simulink model "MF3"  (R2022a)
settings: Solver=VariableStepAuto  StartTime=0.0  StopTime=10.0  RelTol=1e-3
libraries: simulink x8, mbedblockslib x1
settings Model: Creator=FUGAZI  LastModifiedBy=smith

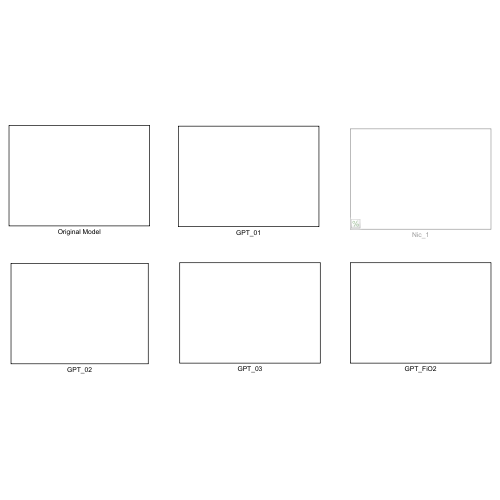
[thumbnail: Simulink's stored preview of the top-level diagram]
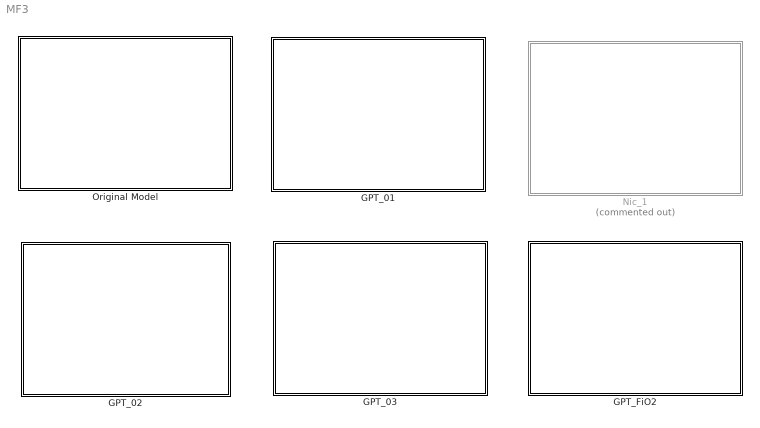
== system MF3 ==
  GPT_01 : Subsystem
  GPT_02 : Subsystem
  GPT_03 : Subsystem
  GPT_FiO2 : Subsystem
  Nic_1 : Subsystem  Commented=on
  Original Model : Subsystem

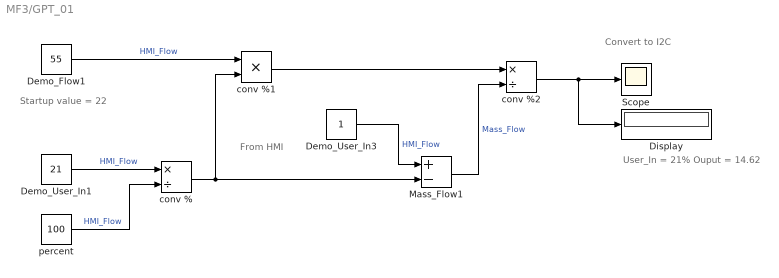
== system MF3/GPT_01 ==
  note: From HMI
  note: Startup value = 22
  note: Convert to I2C
  note: User_In = 21%
      | Ouput = 14.62
  Demo_Flow1 : Constant  Value=55
  Demo_User_In1 : Constant  Value=21
  Demo_User_In3 : Constant
  Display : Display
  Mass_Flow1 : Sum  Inputs=+-
  Scope : Scope
  conv % : Product  Inputs=*/
  conv %1 : Product  Inputs=**
  conv %2 : Product  Inputs=*/
  percent : Constant  Value=100
  wires:
  conv %1/1 -> conv %2/1
  Mass_Flow1/1 -> conv %2/2  "Mass_Flow"
  conv %/1 -> Mass_Flow1/2, conv %1/2
  conv %2/1 -> Display/1, Scope/1
  Demo_Flow1/1 -> conv %1/1  "HMI_Flow"
  Demo_User_In1/1 -> conv %/1  "HMI_Flow"
  percent/1 -> conv %/2  "HMI_Flow"
  Demo_User_In3/1 -> Mass_Flow1/1  "HMI_Flow"

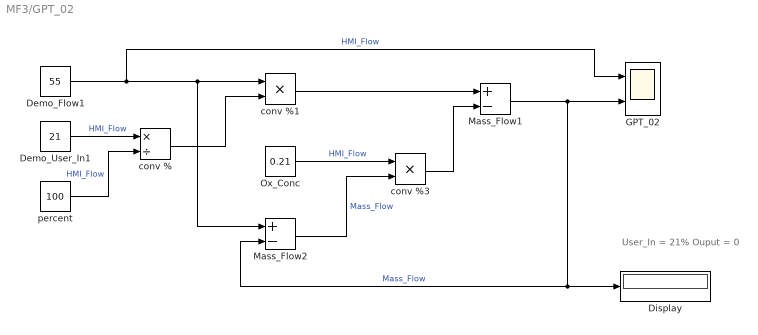
== system MF3/GPT_02 ==
  note: User_In = 21%
      | Ouput = 0
  Demo_Flow1 : Constant  Value=55
  Demo_User_In1 : Constant  Value=21
  Display : Display
  GPT_02 : Scope  NumInputPorts=2
  Mass_Flow1 : Sum  Inputs=+-
  Mass_Flow2 : Sum  Inputs=+-
  Ox_Conc : Constant  Value=0.21
  conv % : Product  Inputs=*/
  conv %1 : Product  Inputs=**
  conv %3 : Product  Inputs=**
  percent : Constant  Value=100
  wires:
  percent/1 -> conv %/2  "HMI_Flow"
  Demo_User_In1/1 -> conv %/1  "HMI_Flow"
  Demo_Flow1/1 -> GPT_02/1, Mass_Flow2/1, conv %1/1  "HMI_Flow"
  conv %/1 -> conv %1/2
  conv %1/1 -> Mass_Flow1/1
  Mass_Flow1/1 -> Display/1, Mass_Flow2/2, GPT_02/2  "Mass_Flow"
  conv %3/1 -> Mass_Flow1/2
  Ox_Conc/1 -> conv %3/1  "HMI_Flow"
  Mass_Flow2/1 -> conv %3/2  "Mass_Flow"

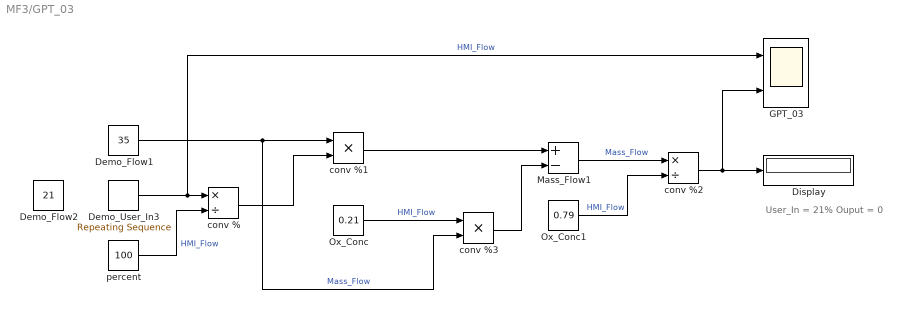
== system MF3/GPT_03 ==
  note: User_In = 21%
      | Ouput = 0
  Demo_Flow1 : Constant  Value=35
  Demo_Flow2 : Constant  Value=21
  Demo_User_In3 : simulink/Sources/Repeating Sequence  rep_seq_t=[0 1 1.1 2 2.1 3 3.1 4 4.1]  rep_seq_y=[21 21 65 65 35 35 45 45 21]
  Display : Display
  GPT_03 : Scope  NumInputPorts=2
  Mass_Flow1 : Sum  Inputs=+-
  Ox_Conc : Constant  Value=0.21
  Ox_Conc1 : Constant  Value=0.79
  conv % : Product  Inputs=*/
  conv %1 : Product  Inputs=**
  conv %2 : Product  Inputs=*/
  conv %3 : Product  Inputs=**
  percent : Constant  Value=100
  wires:
  Demo_Flow1/1 -> conv %3/2, conv %1/1  "Mass_Flow"
  conv %3/1 -> Mass_Flow1/2
  Demo_User_In3/1 -> GPT_03/1, conv %/1  "HMI_Flow"
  Ox_Conc/1 -> conv %3/1  "HMI_Flow"
  percent/1 -> conv %/2  "HMI_Flow"
  conv %1/1 -> Mass_Flow1/1
  conv %/1 -> conv %1/2
  Mass_Flow1/1 -> conv %2/1  "Mass_Flow"
  Ox_Conc1/1 -> conv %2/2  "HMI_Flow"
  conv %2/1 -> GPT_03/2, Display/1

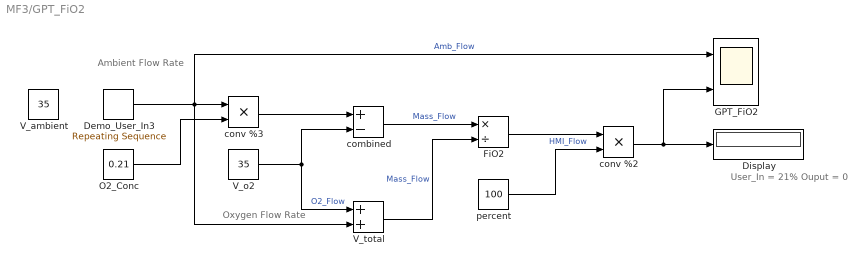
== system MF3/GPT_FiO2 ==
  note: Ambient
      | Flow Rate
  note: User_In = 21%
      | Ouput = 0
  note: Oxygen
      | Flow Rate
  Demo_User_In3 : simulink/Sources/Repeating Sequence  rep_seq_t=[0 1 1.1 2 2.1 3 3.1 4 4.1]  rep_seq_y=[21 21 65 65 35 35 45 45 21]
  Display : Display
  FiO2 : Product  Inputs=*/
  GPT_FiO2 : Scope  NumInputPorts=2
  O2_Conc : Constant  Value=0.21
  V_ambient : Constant  Value=35
  V_o2 : Constant  Value=35
  V_total : Sum
  combined : Sum  Inputs=+-
  conv %2 : Product  Inputs=**
  conv %3 : Product  Inputs=**
  percent : Constant  Value=100
  wires:
  conv %2/1 -> Display/1, GPT_FiO2/2
  O2_Conc/1 -> conv %3/2
  Demo_User_In3/1 -> GPT_FiO2/1, V_total/2, conv %3/1  "Amb_Flow"
  conv %3/1 -> combined/1
  V_o2/1 -> V_total/1, combined/2  "O2_Flow"
  combined/1 -> FiO2/1  "Mass_Flow"
  V_total/1 -> FiO2/2  "Mass_Flow"
  FiO2/1 -> conv %2/1
  percent/1 -> conv %2/2  "HMI_Flow"

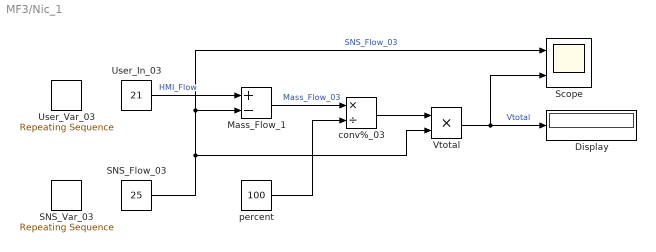
== system MF3/Nic_1 ==
  Display : Display
  Mass_Flow_1 : Sum  Inputs=+-
  SNS_Flow_03 : Constant  Value=25
  SNS_Var_03 : simulink/Sources/Repeating Sequence  rep_seq_t=[0 1 1.1 2 2.1 3 3.1 4 4.1]  rep_seq_y=[21 21 65 65 35 35 45 45 21]
  Scope : Scope  NumInputPorts=2
  User_In_03 : Constant  Value=21
  User_Var_03 : simulink/Sources/Repeating Sequence  rep_seq_t=[0 1 1.1 2 2.1 3 3.1 4 4.1]  rep_seq_y=[21 21 65 65 35 35 45 45 21]
  Vtotal : Product  Inputs=**
  conv%_03 : Product  Inputs=*/
  percent : Constant  Value=100
  wires:
  Vtotal/1 -> Display/1, Scope/2  "Vtotal"
  Mass_Flow_1/1 -> conv%_03/1  "Mass_Flow_03"
  User_In_03/1 -> Mass_Flow_1/1  "HMI_Flow"
  percent/1 -> conv%_03/2
  SNS_Flow_03/1 -> Vtotal/2, Scope/1, Mass_Flow_1/2  "SNS_Flow_03"
  conv%_03/1 -> Vtotal/1

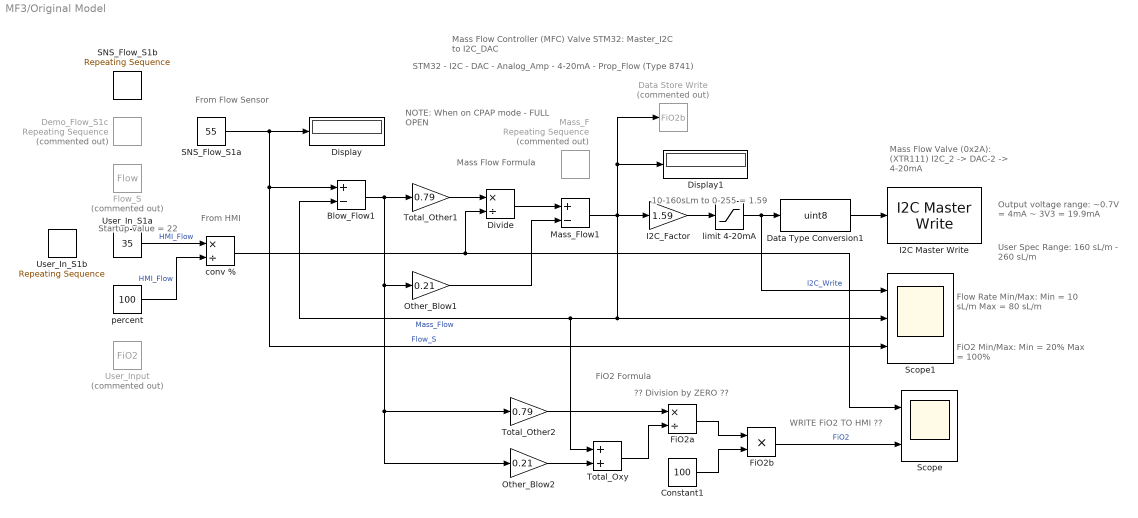
== system MF3/Original Model ==
  note: Startup value = 22
  note: NOTE:
      | When on CPAP mode - FULL OPEN
  note: STM32 - I2C - DAC - Analog_Amp - 4-20mA - Prop_Flow (Type 8741)
  note: FiO2 Formula
  note: Flow Rate Min/Max:
      | Min = 10 sL/m
      | Max = 80 sL/m
  note: Mass Flow Controller (MFC) Valve
      | STM32: Master_I2C to I2C_DAC
  note: FiO2 Min/Max:
      | Min = 20%
      | Max = 100%
  note: Mass Flow Formula
  note: Output voltage range:
      | ~0.7V = 4mA
      | ~ 3V3 = 19.9mA
  note: ?? Division by ZERO ??
  note: WRITE FiO2 TO HMI ??
  note: 10-160sLm to 0-255 = 1.59
  note: From HMI
  note: User Spec Range:
      | 160 sL/m - 260 sL/m
  note: Mass Flow Valve (0x2A):
      | (XTR111)
      | I2C_2 -> DAC-2 -> 4-20mA
  note: From
      | Flow Sensor
  Blow_Flow1 : Sum  Inputs=+-
  Constant1 : Constant  Value=100
  Data Store Write : DataStoreWrite  Commented=on  DataStoreName=FiO2b  IndexOptions=Index vector (dialog)  Indices=1  OutputSizes=1
  Data Type Conversion1 : DataTypeConversion  OutDataTypeStr=uint8  SaturateOnIntegerOverflow=off  RndMeth=Floor
  Demo_Flow_S1c : simulink/Sources/Repeating Sequence  Commented=on  rep_seq_t=[0 1 1.1 2 2.1 3 3.1 4 4.1]  rep_seq_y=[20 20 65 65 35 35 45 45 20]
  Display : Display
  Display1 : Display
  Divide : Product  Inputs=*/
  FiO2a : Product  Inputs=*/
  FiO2b : Product
  Flow_S : DataStoreRead  Commented=on  DataStoreName=Flow  IndexOptions=Index vector (dialog)  Indices=1  OutputSizes=1
  I2C Master Write : mbedblockslib/I2C Master Write  I2CModule=2  Mode=Master  SlaveAddress=uint8(hex2dec('2A'))  SlaveByteOrder=BigEndian  Direction=Transmitter  RegisterAddressMode=on  RegisterAddress=uint8(hex2dec('11'))  SlaveDataType=uint8  DataLength=2  NoAck=off  RepeatedStart=off  OutputStatus=off
      settings: SourceProductBaseCode=MICROBIT,NUCLEO,STMICRODIS
  I2C_Factor : Gain  Gain=1.59
  Mass_F : simulink/Sources/Repeating Sequence  Commented=on  rep_seq_t=[0 1 1.1 2 2.1 3 3.1 4 4.1]  rep_seq_y=[10 10 25 25 50 50 40 40 10]
  Mass_Flow1 : Sum  Inputs=+-
  Other_Blow1 : Gain  Gain=0.21
  Other_Blow2 : Gain  Gain=0.21
  SNS_Flow_S1a : Constant  Value=55
  SNS_Flow_S1b : simulink/Sources/Repeating Sequence  rep_seq_t=[0 1 1.1 2 2.1 3 3.1 4 4.1]  rep_seq_y=[20 20 65 65 35 35 45 45 20]
  Scope : Scope  NumInputPorts=2
  Scope1 : Scope  NumInputPorts=3
  Total_Other1 : Gain  Gain=0.79
  Total_Other2 : Gain  Gain=0.79
  Total_Oxy : Sum
  User_In_S1a : Constant  Value=35
  User_In_S1b : simulink/Sources/Repeating Sequence  rep_seq_t=[0 10 10.1 20 20.1 30 30.1 40 40.1]  rep_seq_y=[21 21 35 35 21 21 35 35 21]
  User_Input : DataStoreRead  Commented=on  DataStoreName=FiO2  IndexOptions=Index vector (dialog)  Indices=1  OutputSizes=1
  conv % : Product  Inputs=*/
  limit 4-20mA : Saturate  UpperLimit=255  LowerLimit=15
  percent : Constant  Value=100
  wires:
  SNS_Flow_S1a/1 -> Display/1, Scope1/3, Blow_Flow1/1  "Flow_S"
  conv %/1 -> Scope/1, Divide/2
  percent/1 -> conv %/2  "HMI_Flow"
  Constant1/1 -> FiO2b/2
  Total_Other1/1 -> Divide/1
  Data Type Conversion1/1 -> I2C Master Write/1
  FiO2a/1 -> FiO2b/1
  limit 4-20mA/1 -> Scope1/1, Data Type Conversion1/1  "I2C_Write"
  I2C_Factor/1 -> limit 4-20mA/1
  Total_Oxy/1 -> FiO2a/2
  Other_Blow1/1 -> Mass_Flow1/2
  FiO2b/1 -> Scope/2  "FiO2"
  Divide/1 -> Mass_Flow1/1
  Total_Other2/1 -> FiO2a/1
  Blow_Flow1/1 -> Other_Blow2/1, Total_Other2/1, Other_Blow1/1, Total_Other1/1
  User_In_S1a/1 -> conv %/1  "HMI_Flow"
  Other_Blow2/1 -> Total_Oxy/2
  Mass_Flow1/1 -> I2C_Factor/1, Total_Oxy/1, Blow_Flow1/2, Scope1/2, Display1/1, Data Store Write/1  "Mass_Flow"
